simulink model "eovsa_corr_300mhz"  (R2012b)
settings: Solver=VariableStepDiscrete  SolverMode=SingleTasking  StartTime=0.0  StopTime=5000  RelTol=1e-3
undefined symbols (not defined in the file or in its folder): A, B, gcbh, PCIN, sfp, xlBlockLoadCallback, xlipgetpartsetting
libraries: xbsIndex_r4 x5996, casper_library_misc x52, simulink x33, dspsigops x24, xps_library x15, casper_library_delays x2
(part 7 of 65)

== system eovsa_corr_300mhz/pfb_fft ==
  note: If this register is not zero, the FFT
      | is overflowing, and you should change
      | the shift shedule to downshift more often.
  fft_shift : Inport
  acc_len : Inport  Port=2
  sync : Inport  Port=3
  adc0_pol0 : Inport  Port=4
  adc0_pol1 : Inport  Port=5
  adc1_pol0 : Inport  Port=6
  adc1_pol1 : Inport  Port=7
  acc_start_skip : Inport  Port=8
  clear_status : Inport  Port=9
  Constant : xbsIndex_r4/Constant  const=0  gui_display_data_type=Fixed-point  arith_type=Unsigned  n_bits=4  bin_pt=0  preci_type=Single  exp_width=8  frac_width=24  explicit_period=on  period=1  equ=P=C  opselect=C  inp2=PCIN>>17  opr=+  inp1=P  carry=CIN  dbl_ovrd=off  block_type=constant
  Convert : xbsIndex_r4/Convert  gui_display_data_type=Fixed-point  arith_type=Unsigned  n_bits=32  bin_pt=0  float_type=Single  exp_bits=8  fraction_bits=24  quantization=Truncate  overflow=Wrap  en=off  latency=0  dbl_ovrd=off  pipeline=off  block_type=convert
      settings: block_version=11.4
  Delay{6..7,12,19..20,24,34,42,47..48} (10 alike) : xbsIndex_r4/Delay  rst=off  infoeditControl=Selection of Reset will increase slice count due to use of real FFs and instead of SRLs  en=off  latency=2  dbl_ovrd=off  reg_retiming=on  block_type=delay
      settings: block_version=11.4
  Register : xbsIndex_r4/Register  init=0  rst=on  en=on  dbl_ovrd=off  block_type=register
  Relational : xbsIndex_r4/Relational  mode=a!=b  en=off  latency=0  dbl_ovrd=off  block_type=relational
  Terminator{10..16} (7 alike) : Terminator
  bus_expand : Subsystem  AncestorBlock=casper_library_flow_control/bus_expand  mask(bus_expand){mode=divisions of equal size, outputNum=4, outputWidth=12, outputBinaryPt=11, outputArithmeticType=1, show_format=off, outputToWorkspace=off, variablePrefix=out, outputToModelAsWell=on}
      mask prompts: outputNum "Number of outputs:"; outputWidth "Output width:"; outputBinaryPt "Output binary point position:"; outputArithmeticType "Output arithmetic type (ufix=0, fix=1, bool=2):"; show_format "Print format string?"; outputToWorkspace "Output to workspace?"; variablePrefix "Variable name prefix:"; outputToModelAsWell "Output to model as well?"
      mask help:
      | Expands a 'bus' made using a bus_create or Xilinx
      | concat block.
      | The input will be divided into the specified number
      | of outputs with the specified arithmetic types.
      | Divisions are made from most significant bit.
      mask init: same as eovsa_corr_300mhz/bus_expand7
      settings: AttributesFormatString=4 outputs
      mask TypeOptions mode: divisions of equal size | divisions of arbitrary size
      mask Callback mode: bus_expand_callback();
      mask Callback outputWidth: bus_expand_callback();
      mask Callback outputToWorkspace: bus_expand_callback();
  bus_expand1 : Subsystem  AncestorBlock=casper_library_flow_control/bus_expand  mask(bus_expand){mode=divisions of equal size, outputNum=4, outputWidth=12, outputBinaryPt=11, outputArithmeticType=1, show_format=off, outputToWorkspace=off, variablePrefix=out, outputToModelAsWell=on}
      mask prompts: outputNum "Number of outputs:"; outputWidth "Output width:"; outputBinaryPt "Output binary point position:"; outputArithmeticType "Output arithmetic type (ufix=0, fix=1, bool=2):"; show_format "Print format string?"; outputToWorkspace "Output to workspace?"; variablePrefix "Variable name prefix:"; outputToModelAsWell "Output to model as well?"
      mask help:
      | Expands a 'bus' made using a bus_create or Xilinx
      | concat block.
      | The input will be divided into the specified number
      | of outputs with the specified arithmetic types.
      | Divisions are made from most significant bit.
      mask init: same as eovsa_corr_300mhz/bus_expand7
      settings: AttributesFormatString=4 outputs
      mask TypeOptions mode: divisions of equal size | divisions of arbitrary size
      mask Callback mode: bus_expand_callback();
      mask Callback outputWidth: bus_expand_callback();
      mask Callback outputToWorkspace: bus_expand_callback();
  bus_expand2 : Subsystem  AncestorBlock=casper_library_flow_control/bus_expand  mask(bus_expand){mode=divisions of equal size, outputNum=4, outputWidth=12, outputBinaryPt=11, outputArithmeticType=1, show_format=off, outputToWorkspace=off, variablePrefix=out, outputToModelAsWell=on}
      mask prompts: outputNum "Number of outputs:"; outputWidth "Output width:"; outputBinaryPt "Output binary point position:"; outputArithmeticType "Output arithmetic type (ufix=0, fix=1, bool=2):"; show_format "Print format string?"; outputToWorkspace "Output to workspace?"; variablePrefix "Variable name prefix:"; outputToModelAsWell "Output to model as well?"
      mask help:
      | Expands a 'bus' made using a bus_create or Xilinx
      | concat block.
      | The input will be divided into the specified number
      | of outputs with the specified arithmetic types.
      | Divisions are made from most significant bit.
      mask init: same as eovsa_corr_300mhz/bus_expand7
      settings: AttributesFormatString=4 outputs
      mask TypeOptions mode: divisions of equal size | divisions of arbitrary size
      mask Callback mode: bus_expand_callback();
      mask Callback outputWidth: bus_expand_callback();
      mask Callback outputToWorkspace: bus_expand_callback();
  bus_expand3 : Subsystem  AncestorBlock=casper_library_flow_control/bus_expand  mask(bus_expand){mode=divisions of equal size, outputNum=4, outputWidth=12, outputBinaryPt=11, outputArithmeticType=1, show_format=off, outputToWorkspace=off, variablePrefix=out, outputToModelAsWell=on}
      mask prompts: outputNum "Number of outputs:"; outputWidth "Output width:"; outputBinaryPt "Output binary point position:"; outputArithmeticType "Output arithmetic type (ufix=0, fix=1, bool=2):"; show_format "Print format string?"; outputToWorkspace "Output to workspace?"; variablePrefix "Variable name prefix:"; outputToModelAsWell "Output to model as well?"
      mask help:
      | Expands a 'bus' made using a bus_create or Xilinx
      | concat block.
      | The input will be divided into the specified number
      | of outputs with the specified arithmetic types.
      | Divisions are made from most significant bit.
      mask init: same as eovsa_corr_300mhz/bus_expand7
      settings: AttributesFormatString=4 outputs
      mask TypeOptions mode: divisions of equal size | divisions of arbitrary size
      mask Callback mode: bus_expand_callback();
      mask Callback outputWidth: bus_expand_callback();
      mask Callback outputToWorkspace: bus_expand_callback();
  fft_wideband_real : xbsIndex_r4/Black Box  init_code=fft_wideband_real_core_config  sim_method=Inactive  verbose=off  block_type=blackbox2
      settings: block_version=11.4
  overflow : Subsystem  Tag=xps:sw_reg  AncestorBlock=xps_library/software_register  mask(swreg){mode=one value, io_dir=To Processor, io_delay=0, sample_period=1, names=reg, bitwidths=32, arith_types=0, bin_pts=0, sim_port=on, show_format=off}
      mask prompts: io_dir "I/O direction"; io_delay "I/O delay"; sample_period "Sample period"; names "Name:"; bitwidths "Bitwidth:"; arith_types "Type (ufix=0, fix=1, bool=2):"; bin_pts "Binary pt:"; sim_port "Provide sim input/output?"; show_format "Print format string?"
      mask init:
      | swreg_init(gcb)
      settings: AttributesFormatString=1output
      mask TypeOptions mode: one value | fields of equal size | fields of arbitrary size
      mask Callback mode: swreg_cb(gcb);
      mask TypeOptions io_dir: To Processor | From Processor
      mask Callback io_dir:
      | mask_enables = get_param(gcb, 'MaskEnables');
      | mask_names = get_param(gcb, 'MaskNames');
      | if strcmp(get_param(gcb, 'io_dir'), 'To Processor'),
      |     mask_enables{ismember(mask_names, 'sample_period')} = 'off';
      | else
      |     mask_enables{ismember(mask_names, 'sample_period')} = 'on';
      | end
      | set_param(gcb, 'MaskEnables', mask_enables);
      mask Callback bitwidths:
      | swreg_maskcheck(gcb);
      | % blk = gcb;
      | % mode = get_param(blk, 'mode');
      | % current_widths = eval(get_param(blk, 'bitwidths'));
      | % if (strcmp(mode, 'one value') || strcmp(mode, 'fields of equal size')) && (length(current_widths) > 1),
      | %     error('Only one width may be specified for this mode.');
      | % elseif strcmp(mode, 'fields of arbitrary size')
      | %     current_names = textscan(strtrim(strrep(strrep(get_param(blk, 'names'), ']', ''), '[', '')), '%s');
      | %     current_names = current_names{1};
      | %     numios = length(current_names);
      | %     if length(current_widths) ~= numios,
      | %         error('%d field names specified, but %d widths?', numios, length(current_widths));
      | %     end
      | % end
      | % total_width = 0;
      | % for ctr = 1 : length(current_widths),
      | %     total_width = total_width + current_widths(ctr);
      | % end
      | % if total_width > 32,
      | %     error('Total width must be 32 or less, set to %d.', total_width);
      | % end
      mask Callback arith_types:
      | [numios, ~, ~, ~, current_types] = swreg_maskcheck(gcb);
      | % blk = gcb;
      | % mode = get_param(blk, 'mode');
      | % current_types = eval(get_param(blk, 'arith_types'));
      | % numios = length(current_types);
      | % if (strcmp(mode, 'one value') || strcmp(mode, 'fields of equal size')) && (length(current_types) > 1),
      | %     error('Only one type may be specified for this mode.');
      | % elseif strcmp(mode, 'fields of arbitrary size')
      | %     current_names = textscan(strtrim(strrep(strrep(get_param(blk, 'names'), ']', ''), '[', '')), '%s');
      | %     current_names = current_names{1};
      | %     numios = length(current_names);
      | %     if length(current_types) ~= numios,
      | %         error('%d field names specified, but %d types?', numios, length(current_types));
      | %     end
      | % end
      | problem = 0;
      | for ctr = 1 : numios,
      |     t = current_types(ctr);
      |     if (t < 0) || (t > 2),
      |         problem = t;
      |         ctr = numios + 1;
      |     end
      | end
      | if problem ~= 0,
      |     error('Type cannot be %i, must be 0, 1 or 2.', problem);
      | end
      mask Callback bin_pts:
      | swreg_maskcheck(gcb);
      | % blk = gcb;
      | % mode = get_param(blk, 'mode');
      | % current_bins = eval(get_param(blk, 'bin_pts'));
      | % if (strcmp(mode, 'one value') || strcmp(mode, 'fields of equal size')) && (length(current_bins) > 1),
      | %     error('Only one binary pt may be specified for this mode.');
      | % elseif strcmp(mode, 'fields of arbitrary size')
      | %     current_names = textscan(strtrim(strrep(strrep(get_param(blk, 'names'), ']', ''), '[', '')), '%s');
      | %     current_names = current_names{1};
      | %     numios = length(current_names);
      | %     if length(current_bins) ~= numios,
      | %         error('%d field names specified, but %d binary pts?', numios, length(current_bins));
      | %     end
      | % end
  pfb_fir_real : xbsIndex_r4/Black Box  init_code=pfb_fir_4input_core_config  sim_method=Inactive  verbose=off  block_type=blackbox2
      settings: block_version=11.4
  power_td1 : Subsystem
  power_td2 : Subsystem
  power_td3 : Subsystem
  power_td4 : Subsystem
  sync_out0 : Outport
  x0_out0 : Outport  Port=2
  x0_out1 : Outport  Port=3
  y0_out0 : Outport  Port=4
  y0_out1 : Outport  Port=5
  x1_out0 : Outport  Port=6
  x1_out1 : Outport  Port=7
  y1_out0 : Outport  Port=8
  y1_out1 : Outport  Port=9
  adc0_pol0_P : Outport  Port=10
  adc0_pol0_P2 : Outport  Port=11
  adc0_pol1_P : Outport  Port=12
  adc0_pol1_P2 : Outport  Port=13
  adc1_pol0_P : Outport  Port=14
  adc1_pol0_P2 : Outport  Port=15
  adc1_pol1_P : Outport  Port=16
  adc1_pol1_P2 : Outport  Port=17
  acc_num : Outport  Port=18
  acc_valid : Outport  Port=19
  wires:
  power_td1/2(P) -> Delay47/1
  power_td1/3(P2) -> Delay48/1
  power_td1/4(acc_valid) -> Delay34/1
  [acc_start_skip] -> power_td1/4(acc_start_skip)
  acc_len/1 -> [acc_len]
  fft_wideband_real/10 -> Relational/1, Terminator13/1
  Relational/1 -> Register/3, Register/1
  Constant/1 -> Relational/2
  Register/1 -> Convert/1
  clear_status/1 -> Register/2
  Convert/1 -> overflow/1(out_reg)
  fft_shift/1 -> fft_wideband_real/2
  acc_start_skip/1 -> [acc_start_skip]
  sync/1 -> [sync], pfb_fir_real/1
  adc0_pol0/1 -> power_td1/2(din), pfb_fir_real/2
  adc0_pol1/1 -> power_td2/2(din), pfb_fir_real/3
  adc1_pol0/1 -> power_td3/2(din), pfb_fir_real/4
  adc1_pol1/1 -> power_td4/2(din), pfb_fir_real/5
  [acc_len] -> power_td1/3(acc_len)
  [sync] -> power_td1/1(sync)
  power_td2/2(P) -> Delay6/1
  power_td2/3(P2) -> Delay7/1
  power_td2/1(acc_num) -> Terminator10/1
  power_td2/4(acc_valid) -> Terminator11/1
  [acc_start_skip] -> power_td2/4(acc_start_skip)
  [acc_len] -> power_td2/3(acc_len)
  Delay6/1 -> adc0_pol1_P/1
  Delay7/1 -> adc0_pol1_P2/1
  [sync] -> power_td2/1(sync)
  power_td3/2(P) -> Delay12/1
  power_td3/3(P2) -> Delay19/1
  power_td3/1(acc_num) -> Terminator12/1
  power_td3/4(acc_valid) -> Terminator14/1
  [acc_start_skip] -> power_td3/4(acc_start_skip)
  [acc_len] -> power_td3/3(acc_len)
  [sync] -> power_td3/1(sync)
  power_td4/2(P) -> Delay20/1
  power_td4/3(P2) -> Delay24/1
  power_td4/1(acc_num) -> Terminator15/1
  power_td4/4(acc_valid) -> Terminator16/1
  [acc_start_skip] -> power_td4/4(acc_start_skip)
  [acc_len] -> power_td4/3(acc_len)
  Delay20/1 -> adc1_pol1_P/1
  Delay24/1 -> adc1_pol1_P2/1
  [sync] -> power_td4/1(sync)
  power_td1/1(acc_num) -> Delay42/1
  Delay12/1 -> adc1_pol0_P/1
  Delay19/1 -> adc1_pol0_P2/1
  Delay42/1 -> acc_num/1
  Delay47/1 -> adc0_pol0_P/1
  Delay48/1 -> adc0_pol0_P2/1
  Delay34/1 -> acc_valid/1
  pfb_fir_real/1 -> fft_wideband_real/1
  bus_expand/1(msb_out4) -> fft_wideband_real/3
  bus_expand/3(out2) -> fft_wideband_real/5
  bus_expand/2(out3) -> fft_wideband_real/4
  bus_expand/4(lsb_out1) -> fft_wideband_real/6
  bus_expand1/4(lsb_out1) -> fft_wideband_real/10
  bus_expand1/3(out2) -> fft_wideband_real/9
  bus_expand1/2(out3) -> fft_wideband_real/8
  bus_expand1/1(msb_out4) -> fft_wideband_real/7
  bus_expand2/2(out3) -> fft_wideband_real/12
  bus_expand2/1(msb_out4) -> fft_wideband_real/11
  bus_expand2/4(lsb_out1) -> fft_wideband_real/14
  bus_expand3/3(out2) -> fft_wideband_real/17
  bus_expand2/3(out2) -> fft_wideband_real/13
  bus_expand3/2(out3) -> fft_wideband_real/16
  bus_expand3/4(lsb_out1) -> fft_wideband_real/18
  bus_expand3/1(msb_out4) -> fft_wideband_real/15
  pfb_fir_real/2 -> bus_expand/1(bus_in)
  pfb_fir_real/3 -> bus_expand1/1(bus_in)
  pfb_fir_real/4 -> bus_expand2/1(bus_in)
  pfb_fir_real/5 -> bus_expand3/1(bus_in)
  fft_wideband_real/1 -> sync_out0/1
  fft_wideband_real/2 -> x0_out0/1
  fft_wideband_real/3 -> x0_out1/1
  fft_wideband_real/4 -> y0_out0/1
  fft_wideband_real/5 -> y0_out1/1
  fft_wideband_real/6 -> x1_out0/1
  fft_wideband_real/7 -> x1_out1/1
  fft_wideband_real/8 -> y1_out0/1
  fft_wideband_real/9 -> y1_out1/1

== system eovsa_corr_300mhz/phase_switching ==
  walsh_start : Inport
  phs_ant0 : Inport  Port=2
  phs_ant1 : Inport  Port=3
  adc0_0_0 : Inport  Port=4
  adc0_0_1 : Inport  Port=5
  adc0_0_2 : Inport  Port=6
  adc0_0_3 : Inport  Port=7
  adc0_1_0 : Inport  Port=8
  adc0_1_1 : Inport  Port=9
  adc0_1_2 : Inport  Port=10
  adc0_1_3 : Inport  Port=11
  adc0_sync : Inport  Port=12
  adc0_overflow : Inport  Port=13
  adc1_0_0 : Inport  Port=14
  adc1_0_1 : Inport  Port=15
  adc1_0_2 : Inport  Port=16
  adc1_0_3 : Inport  Port=17
  adc1_1_0 : Inport  Port=18
  adc1_1_1 : Inport  Port=19
  adc1_1_2 : Inport  Port=20
  adc1_1_3 : Inport  Port=21
  adc1_sync : Inport  Port=22
  adc1_overflow : Inport  Port=23
  pps_in : Inport  Port=24
  Delay{1,3..4,7,9,12,14..16,18} (10 alike) : xbsIndex_r4/Delay  rst=off  infoeditControl=Selection of Reset will increase slice count due to use of real FFs and instead of SRLs  en=off  latency=1  dbl_ovrd=off  reg_retiming=on  block_type=delay
  Delay{2,5,8,10..11,13,17} (7 alike) : xbsIndex_r4/Delay  rst=off  infoeditControl=Selection of Reset will increase slice count due to use of real FFs and instead of SRLs  en=off  latency=9  dbl_ovrd=off  reg_retiming=on  block_type=delay
  Delay6 : xbsIndex_r4/Delay  rst=off  infoeditControl=Selection of Reset will increase slice count due to use of real FFs and instead of SRLs  en=off  latency=10  dbl_ovrd=off  reg_retiming=on  block_type=delay
  Mux1 : xbsIndex_r4/Mux  inputs=2  en=off  latency=1  precision=Full  arith_type=Unsigned  n_bits=16  bin_pt=14  quantization=Truncate  overflow=Wrap  dbl_ovrd=off  block_type=mux
      settings: block_version=11.4
  phase_switching_select : Subsystem
  pol_pack0 : Subsystem
  pol_pack1 : Subsystem
  pol_pack2 : Subsystem
  pol_pack3 : Subsystem
  sync_out : Outport
  adc0_pol0 : Outport  Port=2
  adc0_pol1 : Outport  Port=3
  adc_sync : Outport  Port=4
  adc0_overflow_out : Outport  Port=5
  adc1_pol0 : Outport  Port=6
  adc1_pol1 : Outport  Port=7
  adc1_overflow_out : Outport  Port=8
  wires:
  pol_pack0/1(Out) -> Delay1/1
  pol_pack3/1(Out) -> Delay4/1
  phase_switching_select/2(phs_val_ant0) -> pol_pack0/1(phase), pol_pack3/1(phase)
  walsh_start/1 -> phase_switching_select/1(walsh_start)
  phase_switching_select/1(sync_out) -> Delay16/1
  Delay16/1 -> Delay15/1
  adc0_0_0/1 -> pol_pack0/2(In1)
  adc0_0_1/1 -> pol_pack0/3(In2)
  adc0_0_2/1 -> pol_pack0/4(In3)
  adc0_0_3/1 -> pol_pack0/5(In4)
  adc0_1_0/1 -> pol_pack3/2(In1)
  adc0_1_1/1 -> pol_pack3/3(In2)
  adc0_1_2/1 -> pol_pack3/4(In3)
  adc0_1_3/1 -> pol_pack3/5(In4)
  adc0_overflow/1 -> Delay3/1
  Delay3/1 -> Delay12/1
  pol_pack1/1(Out) -> Delay14/1
  pol_pack2/1(Out) -> Delay18/1
  phase_switching_select/3(phs_val_ant1) -> pol_pack2/1(phase), pol_pack1/1(phase)
  adc1_0_0/1 -> pol_pack1/2(In1)
  adc1_0_1/1 -> pol_pack1/3(In2)
  adc1_0_2/1 -> pol_pack1/4(In3)
  adc1_0_3/1 -> pol_pack1/5(In4)
  adc1_1_0/1 -> pol_pack2/2(In1)
  adc1_1_1/1 -> pol_pack2/3(In2)
  adc1_1_2/1 -> pol_pack2/4(In3)
  adc1_1_3/1 -> pol_pack2/5(In4)
  adc1_overflow/1 -> Delay7/1
  Delay7/1 -> Delay6/1
  Delay15/1 -> Delay8/1
  Delay6/1 -> adc1_overflow_out/1
  phs_ant0/1 -> phase_switching_select/2(ant_0_seq)
  phs_ant1/1 -> phase_switching_select/3(ant_1_seq)
  adc0_sync/1 -> Mux1/2
  adc1_sync/1 -> Mux1/3
  Mux1/1 -> Delay9/1
  Delay8/1 -> sync_out/1
  Delay1/1 -> Delay2/1
  Delay2/1 -> adc0_pol0/1
  Delay4/1 -> Delay5/1
  Delay5/1 -> adc0_pol1/1
  Delay9/1 -> Delay10/1
  Delay10/1 -> adc_sync/1
  Delay12/1 -> Delay11/1
  Delay11/1 -> adc0_overflow_out/1
  Delay14/1 -> Delay13/1
  Delay13/1 -> adc1_pol0/1
  Delay18/1 -> Delay17/1
  Delay17/1 -> adc1_pol1/1
  pps_in/1 -> Mux1/1

== system eovsa_corr_300mhz/pipeline21 ==
  d : Inport
  Register0 : xbsIndex_r4/Register  init=0  rst=off  en=off  dbl_ovrd=off  block_type=register
      settings: block_version=11.4
  q : Outport
  wires:
  d/1 -> Register0/1
  Register0/1 -> q/1

== system eovsa_corr_300mhz/pkt_gate ==
  rst_i : Inport
  data_i : Inport  Port=2
  dv_i : Inport  Port=3
  ip_i : Inport  Port=4
  port_i : Inport  Port=5
  eof_i : Inport  Port=6
  Delay25 : xbsIndex_r4/Delay  rst=off  infoeditControl=Selection of Reset will increase slice count due to use of real FFs and instead of SRLs  en=off  latency=1  dbl_ovrd=off  reg_retiming=off  block_type=delay
      settings: block_version=11.4
  Delay26 : xbsIndex_r4/Delay  rst=off  infoeditControl=Selection of Reset will increase slice count due to use of real FFs and instead of SRLs  en=off  latency=1  dbl_ovrd=off  reg_retiming=off  block_type=delay
      settings: block_version=11.4
  Delay27 : xbsIndex_r4/Delay  rst=off  infoeditControl=Selection of Reset will increase slice count due to use of real FFs and instead of SRLs  en=off  latency=1  dbl_ovrd=off  reg_retiming=on  block_type=delay
      settings: block_version=11.4
  Delay48 : xbsIndex_r4/Delay  rst=off  infoeditControl=Selection of Reset will increase slice count due to use of real FFs and instead of SRLs  en=off  latency=1  dbl_ovrd=off  reg_retiming=on  block_type=delay
      settings: block_version=11.4
  Delay49 : xbsIndex_r4/Delay  rst=off  infoeditControl=Selection of Reset will increase slice count due to use of real FFs and instead of SRLs  en=off  latency=1  dbl_ovrd=off  reg_retiming=on  block_type=delay
      settings: block_version=11.4
  Logical12 : xbsIndex_r4/Logical  logical_function=AND  inputs=2  en=off  latency=1  precision=Full  arith_type=Unsigned  n_bits=16  bin_pt=0  align_bp=on  dbl_ovrd=off  block_type=logical
  Register : xbsIndex_r4/Register  init=0  rst=off  en=on  dbl_ovrd=off  block_type=register
  rst_o : Outport
  data_o : Outport  Port=2
  dv_o : Outport  Port=3
  ip_o : Outport  Port=4
  port_o : Outport  Port=5
  eof_o : Outport  Port=6
  wires:
  rst_i/1 -> Delay26/1
  Delay26/1 -> rst_o/1
  Delay27/1 -> data_o/1
  data_i/1 -> Delay27/1
  port_i/1 -> Delay49/1
  eof_i/1 -> Register/2, Delay25/1
  dv_i/1 -> Logical12/2
  Delay49/1 -> port_o/1
  Delay25/1 -> eof_o/1
  ip_i/1 -> Delay48/1
  Logical12/1 -> dv_o/1
  Delay48/1 -> ip_o/1
  [ten_gbe_en] -> Register/1
  Register/1 -> Logical12/1

== system eovsa_corr_300mhz/pkt_gate1 ==
  rst_i : Inport
  data_i : Inport  Port=2
  dv_i : Inport  Port=3
  ip_i : Inport  Port=4
  port_i : Inport  Port=5
  eof_i : Inport  Port=6
  Delay{25..27,49} (4 alike) : xbsIndex_r4/Delay  rst=off  infoeditControl=Selection of Reset will increase slice count due to use of real FFs and instead of SRLs  en=off  latency=3  dbl_ovrd=off  reg_retiming=on  block_type=delay
      settings: block_version=11.4
  Delay48 : xbsIndex_r4/Delay  rst=off  infoeditControl=Selection of Reset will increase slice count due to use of real FFs and instead of SRLs  en=off  latency=0  dbl_ovrd=off  reg_retiming=on  block_type=delay
      settings: block_version=11.4
  Logical12 : xbsIndex_r4/Logical  logical_function=AND  inputs=2  en=off  latency=3  precision=Full  arith_type=Unsigned  n_bits=16  bin_pt=0  align_bp=on  dbl_ovrd=off  block_type=logical
  Register : xbsIndex_r4/Register  init=0  rst=off  en=on  dbl_ovrd=off  block_type=register
  rst_o : Outport
  data_o : Outport  Port=2
  dv_o : Outport  Port=3
  ip_o : Outport  Port=4
  port_o : Outport  Port=5
  eof_o : Outport  Port=6
  wires:
  rst_i/1 -> Delay26/1
  Delay26/1 -> rst_o/1
  Delay27/1 -> data_o/1
  data_i/1 -> Delay27/1
  port_i/1 -> Delay49/1
  eof_i/1 -> Register/2, Delay25/1
  dv_i/1 -> Logical12/2
  Delay49/1 -> port_o/1
  Delay25/1 -> eof_o/1
  ip_i/1 -> Delay48/1
  Logical12/1 -> dv_o/1
  Delay48/1 -> ip_o/1
  Register/1 -> Logical12/1
  [ten_gbe_en] -> Register/1

== system eovsa_corr_300mhz/pkt_gate2 ==
  rst_i : Inport
  data_i : Inport  Port=2
  dv_i : Inport  Port=3
  ip_i : Inport  Port=4
  port_i : Inport  Port=5
  eof_i : Inport  Port=6
  Delay{25..27,49} (4 alike) : xbsIndex_r4/Delay  rst=off  infoeditControl=Selection of Reset will increase slice count due to use of real FFs and instead of SRLs  en=off  latency=3  dbl_ovrd=off  reg_retiming=on  block_type=delay
      settings: block_version=11.4
  Delay48 : xbsIndex_r4/Delay  rst=off  infoeditControl=Selection of Reset will increase slice count due to use of real FFs and instead of SRLs  en=off  latency=0  dbl_ovrd=off  reg_retiming=on  block_type=delay
      settings: block_version=11.4
  Logical12 : xbsIndex_r4/Logical  logical_function=AND  inputs=2  en=off  latency=3  precision=Full  arith_type=Unsigned  n_bits=16  bin_pt=0  align_bp=on  dbl_ovrd=off  block_type=logical
  Register : xbsIndex_r4/Register  init=0  rst=off  en=on  dbl_ovrd=off  block_type=register
  rst_o : Outport
  data_o : Outport  Port=2
  dv_o : Outport  Port=3
  ip_o : Outport  Port=4
  port_o : Outport  Port=5
  eof_o : Outport  Port=6
  wires:
  [ten_gbe_en] -> Register/1
  Register/1 -> Logical12/1
  Delay48/1 -> ip_o/1
  Logical12/1 -> dv_o/1
  ip_i/1 -> Delay48/1
  Delay25/1 -> eof_o/1
  Delay49/1 -> port_o/1
  dv_i/1 -> Logical12/2
  eof_i/1 -> Delay25/1, Register/2
  port_i/1 -> Delay49/1
  data_i/1 -> Delay27/1
  Delay27/1 -> data_o/1
  Delay26/1 -> rst_o/1
  rst_i/1 -> Delay26/1

== system eovsa_corr_300mhz/pkt_gate3 ==
  rst_i : Inport
  data_i : Inport  Port=2
  dv_i : Inport  Port=3
  ip_i : Inport  Port=4
  port_i : Inport  Port=5
  eof_i : Inport  Port=6
  Delay{25..27,48..49} (5 alike) : xbsIndex_r4/Delay  rst=off  infoeditControl=Selection of Reset will increase slice count due to use of real FFs and instead of SRLs  en=off  latency=1  dbl_ovrd=off  reg_retiming=on  block_type=delay
      settings: block_version=11.4
  Logical12 : xbsIndex_r4/Logical  logical_function=AND  inputs=2  en=off  latency=1  precision=Full  arith_type=Unsigned  n_bits=16  bin_pt=0  align_bp=on  dbl_ovrd=off  block_type=logical
  Register : xbsIndex_r4/Register  init=0  rst=off  en=on  dbl_ovrd=off  block_type=register
  rst_o : Outport
  data_o : Outport  Port=2
  dv_o : Outport  Port=3
  ip_o : Outport  Port=4
  port_o : Outport  Port=5
  eof_o : Outport  Port=6
  wires:
  rst_i/1 -> Delay26/1
  Delay26/1 -> rst_o/1
  Delay27/1 -> data_o/1
  data_i/1 -> Delay27/1
  port_i/1 -> Delay49/1
  eof_i/1 -> Register/2, Delay25/1
  dv_i/1 -> Logical12/2
  Delay49/1 -> port_o/1
  Delay25/1 -> eof_o/1
  ip_i/1 -> Delay48/1
  Logical12/1 -> dv_o/1
  Delay48/1 -> ip_o/1
  Register/1 -> Logical12/1
  [ten_gbe_en] -> Register/1

== system eovsa_corr_300mhz/pol_snap ==
  note: Generate stop
      | when in circular
      | capture mode
  note: Delay start
      | of capture
  note: ctrl:
      | bit0: Put a posedge here
      |         to enable a new capture.
      | bit1: ignore external trigger
      |         and trigger immediately.
      | bit2: ignore external write
      |         enable and capture on
      |         every FPGA clock.
      | bit3: continuously capture
      |         data until we get an
      |         external stop command.
  note: Offset in vector
      | from first element
      | captured, used
      | during circular capture
  note: Number of
      | bytes in
      | buffer and
      | done bit
  note: Number of valid
      | data samples to
      | skip after trigger
      | before starting
      | capture
  note: Value on vin
      | aligned with
      | first sample on
      | din captured
  din : Inport
  we : Inport  Port=2
  trig : Inport  Port=3
  add_del : xbsIndex_r4/Delay  rst=off  infoeditControl=Selection of Reset will increase slice count due to use of real FFs and instead of SRLs  en=off  latency=1  dbl_ovrd=off  reg_retiming=on  block_type=delay
      settings: block_version=11.4
  add_gen : Subsystem  AncestorBlock=casper_library_scopes/snapshot/add_gen  mask{counter_size=11+3+1, increment=8, nsamples=11, burst_size=0, use_dsp48=on}
      mask prompts: counter_size "Address counter size (2^?)"; increment "Address counter increment"; nsamples "Number of samples (2^?)"; burst_size "Burst size (2^?)"; use_dsp48 "dsp48 counter/s"
      mask init:
      | set_param(gcb,'LinkStatus','inactive');
      | if strcmp(use_dsp48,'on'),
      |     set_param([gcb,'/add_gen'],'implementation','DSP48');
      | else
      |     set_param([gcb,'/add_gen'],'implementation','Fabric');
      | end
  basic_ctrl : Subsystem  AncestorBlock=casper_library_scopes/snapshot/basic_ctrl  mask{dram=off, data_width=64}
      mask prompts: data_width "data width"
  bram : Subsystem  Tag=xps:bram  AncestorBlock=xps_library/Shared BRAM  mask{arith_type=Unsigned, addr_width=11, data_width=64, reg_prim_output=on, reg_core_output=on, optimization=Minimum_Area, data_bin_pt=0, init_vals=[0:2^10-1], sample_rate=1}
      mask prompts: arith_type "Output Data Type"; addr_width "Address width"; data_width "Data Width"; reg_prim_output "Register Primitive Output"; reg_core_output "Register Core Output"; data_bin_pt "Data Binary Point"; init_vals "Initial values (simulation only)"; sample_rate "Sample rate"
      mask init:
      | shared_bram_mask;
      mask TypeOptions arith_type: Unsigned | Signed  (2's comp)
      mask TypeOptions data_width: 8 | 16 | 32 | 64 | 128
      mask TypeOptions optimization: Minimum_Area | Low_Power
  cast : xbsIndex_r4/Convert  gui_display_data_type=Fixed-point  arith_type=Unsigned  n_bits=64  bin_pt=0  float_type=Single  exp_bits=8  fraction_bits=24  quantization=Truncate  overflow=Wrap  en=off  latency=0  dbl_ovrd=off  pipeline=off  block_type=convert
      settings: block_version=11.4
  const0 : Constant  Value=0
  ctrl : Subsystem  Tag=xps:sw_reg  AncestorBlock=xps_library/software_register  mask(swreg){mode=one value, io_dir=From Processor, io_delay=0, sample_period=1, names=reg, bitwidths=32, arith_types=0, bin_pts=0, sim_port=on, show_format=off}
      mask prompts: io_dir "I/O direction"; io_delay "I/O delay"; sample_period "Sample period"; names "Name:"; bitwidths "Bitwidth:"; arith_types "Type (ufix=0, fix=1, bool=2):"; bin_pts "Binary pt:"; sim_port "Provide sim input/output?"; show_format "Print format string?"
      mask init:
      | swreg_init(gcb)
      settings: AttributesFormatString=1input
      mask TypeOptions mode: one value | fields of equal size | fields of arbitrary size
      mask Callback mode: swreg_cb(gcb);
      mask TypeOptions io_dir: To Processor | From Processor
      mask Callback io_dir:
      | mask_enables = get_param(gcb, 'MaskEnables');
      | mask_names = get_param(gcb, 'MaskNames');
      | if strcmp(get_param(gcb, 'io_dir'), 'To Processor'),
      |     mask_enables{ismember(mask_names, 'sample_period')} = 'off';
      | else
      |     mask_enables{ismember(mask_names, 'sample_period')} = 'on';
      | end
      | set_param(gcb, 'MaskEnables', mask_enables);
      mask Callback bitwidths:
      | swreg_maskcheck(gcb);
      | % blk = gcb;
      | % mode = get_param(blk, 'mode');
      | % current_widths = eval(get_param(blk, 'bitwidths'));
      | % if (strcmp(mode, 'one value') || strcmp(mode, 'fields of equal size')) && (length(current_widths) > 1),
      | %     error('Only one width may be specified for this mode.');
      | % elseif strcmp(mode, 'fields of arbitrary size')
      | %     current_names = textscan(strtrim(strrep(strrep(get_param(blk, 'names'), ']', ''), '[', '')), '%s');
      | %     current_names = current_names{1};
      | %     numios = length(current_names);
      | %     if length(current_widths) ~= numios,
      | %         error('%d field names specified, but %d widths?', numios, length(current_widths));
      | %     end
      | % end
      | % total_width = 0;
      | % for ctr = 1 : length(current_widths),
      | %     total_width = total_width + current_widths(ctr);
      | % end
      | % if total_width > 32,
      | %     error('Total width must be 32 or less, set to %d.', total_width);
      | % end
      mask Callback arith_types:
      | [numios, ~, ~, ~, current_types] = swreg_maskcheck(gcb);
      | % blk = gcb;
      | % mode = get_param(blk, 'mode');
      | % current_types = eval(get_param(blk, 'arith_types'));
      | % numios = length(current_types);
      | % if (strcmp(mode, 'one value') || strcmp(mode, 'fields of equal size')) && (length(current_types) > 1),
      | %     error('Only one type may be specified for this mode.');
      | % elseif strcmp(mode, 'fields of arbitrary size')
      | %     current_names = textscan(strtrim(strrep(strrep(get_param(blk, 'names'), ']', ''), '[', '')), '%s');
      | %     current_names = current_names{1};
      | %     numios = length(current_names);
      | %     if length(current_types) ~= numios,
      | %         error('%d field names specified, but %d types?', numios, length(current_types));
      | %     end
      | % end
      | problem = 0;
      | for ctr = 1 : numios,
      |     t = current_types(ctr);
      |     if (t < 0) || (t > 2),
      |         problem = t;
      |         ctr = numios + 1;
      |     end
      | end
      | if problem ~= 0,
      |     error('Type cannot be %i, must be 0, 1 or 2.', problem);
      | end
      mask Callback bin_pts:
      | swreg_maskcheck(gcb);
      | % blk = gcb;
      | % mode = get_param(blk, 'mode');
      | % current_bins = eval(get_param(blk, 'bin_pts'));
      | % if (strcmp(mode, 'one value') || strcmp(mode, 'fields of equal size')) && (length(current_bins) > 1),
      | %     error('Only one binary pt may be specified for this mode.');
      | % elseif strcmp(mode, 'fields of arbitrary size')
      | %     current_names = textscan(strtrim(strrep(strrep(get_param(blk, 'names'), ']', ''), '[', '')), '%s');
      | %     current_names = current_names{1};
      | %     numios = length(current_names);
      | %     if length(current_bins) ~= numios,
      | %         error('%d field names specified, but %d binary pts?', numios, length(current_bins));
      | %     end
      | % end
  dat_del : xbsIndex_r4/Delay  rst=off  infoeditControl=Selection of Reset will increase slice count due to use of real FFs and instead of SRLs  en=off  latency=1  dbl_ovrd=off  reg_retiming=off  block_type=delay
      settings: block_version=11.4
  g_tr_en_cnt : Terminator
  gbram : Terminator
  gstatus : Terminator
  gval : Terminator
  never : xbsIndex_r4/Constant  const=0  gui_display_data_type=Fixed-point  arith_type=Boolean  n_bits=16  bin_pt=14  preci_type=Single  exp_width=8  frac_width=24  explicit_period=on  period=1  equ=P=C  opselect=C  inp2=PCIN>>17  opr=+  inp1=P  carry=CIN  dbl_ovrd=off  block_type=constant
  ri : xbsIndex_r4/Reinterpret  force_arith_type=on  arith_type=Unsigned  force_bin_pt=on  bin_pt=0  block_type=reinterpret
      settings: infoedit="Changes signal type without altering the binary representation.   You can changed the signal between signed and unsigned, and relocate the binary point.<br><br>Hardware notes: In hardware this block costs nothing.<br><br>Example:  Suppose the input is 6 bits wide, signed, with 2 fractional bits, and the output is forced to unsigned with 0 fractional bits.  Then an input of -2.0 (1110.00 in binary 2's complement) becomes an output of 56 (111000 in binary)."
  status : Subsystem  Tag=xps:sw_reg  AncestorBlock=xps_library/software_register  mask(swreg){mode=one value, io_dir=To Processor, io_delay=0, sample_period=1, names=reg, bitwidths=32, arith_types=0, bin_pts=0, sim_port=on, show_format=off}
      mask prompts: io_dir "I/O direction"; io_delay "I/O delay"; sample_period "Sample period"; names "Name:"; bitwidths "Bitwidth:"; arith_types "Type (ufix=0, fix=1, bool=2):"; bin_pts "Binary pt:"; sim_port "Provide sim input/output?"; show_format "Print format string?"
      mask init:
      | swreg_init(gcb)
      settings: AttributesFormatString=1output
      mask TypeOptions mode: one value | fields of equal size | fields of arbitrary size
      mask Callback mode: swreg_cb(gcb);
      mask TypeOptions io_dir: To Processor | From Processor
      mask Callback io_dir:
      | mask_enables = get_param(gcb, 'MaskEnables');
      | mask_names = get_param(gcb, 'MaskNames');
      | if strcmp(get_param(gcb, 'io_dir'), 'To Processor'),
      |     mask_enables{ismember(mask_names, 'sample_period')} = 'off';
      | else
      |     mask_enables{ismember(mask_names, 'sample_period')} = 'on';
      | end
      | set_param(gcb, 'MaskEnables', mask_enables);
      mask Callback bitwidths:
      | swreg_maskcheck(gcb);
      | % blk = gcb;
      | % mode = get_param(blk, 'mode');
      | % current_widths = eval(get_param(blk, 'bitwidths'));
      | % if (strcmp(mode, 'one value') || strcmp(mode, 'fields of equal size')) && (length(current_widths) > 1),
      | %     error('Only one width may be specified for this mode.');
      | % elseif strcmp(mode, 'fields of arbitrary size')
      | %     current_names = textscan(strtrim(strrep(strrep(get_param(blk, 'names'), ']', ''), '[', '')), '%s');
      | %     current_names = current_names{1};
      | %     numios = length(current_names);
      | %     if length(current_widths) ~= numios,
      | %         error('%d field names specified, but %d widths?', numios, length(current_widths));
      | %     end
      | % end
      | % total_width = 0;
      | % for ctr = 1 : length(current_widths),
      | %     total_width = total_width + current_widths(ctr);
      | % end
      | % if total_width > 32,
      | %     error('Total width must be 32 or less, set to %d.', total_width);
      | % end
      mask Callback arith_types:
      | [numios, ~, ~, ~, current_types] = swreg_maskcheck(gcb);
      | % blk = gcb;
      | % mode = get_param(blk, 'mode');
      | % current_types = eval(get_param(blk, 'arith_types'));
      | % numios = length(current_types);
      | % if (strcmp(mode, 'one value') || strcmp(mode, 'fields of equal size')) && (length(current_types) > 1),
      | %     error('Only one type may be specified for this mode.');
      | % elseif strcmp(mode, 'fields of arbitrary size')
      | %     current_names = textscan(strtrim(strrep(strrep(get_param(blk, 'names'), ']', ''), '[', '')), '%s');
      | %     current_names = current_names{1};
      | %     numios = length(current_names);
      | %     if length(current_types) ~= numios,
      | %         error('%d field names specified, but %d types?', numios, length(current_types));
      | %     end
      | % end
      | problem = 0;
      | for ctr = 1 : numios,
      |     t = current_types(ctr);
      |     if (t < 0) || (t > 2),
      |         problem = t;
      |         ctr = numios + 1;
      |     end
      | end
      | if problem ~= 0,
      |     error('Type cannot be %i, must be 0, 1 or 2.', problem);
      | end
      mask Callback bin_pts:
      | swreg_maskcheck(gcb);
      | % blk = gcb;
      | % mode = get_param(blk, 'mode');
      | % current_bins = eval(get_param(blk, 'bin_pts'));
      | % if (strcmp(mode, 'one value') || strcmp(mode, 'fields of equal size')) && (length(current_bins) > 1),
      | %     error('Only one binary pt may be specified for this mode.');
      | % elseif strcmp(mode, 'fields of arbitrary size')
      | %     current_names = textscan(strtrim(strrep(strrep(get_param(blk, 'names'), ']', ''), '[', '')), '%s');
      | %     current_names = current_names{1};
      | %     numios = length(current_names);
      | %     if length(current_bins) ~= numios,
      | %         error('%d field names specified, but %d binary pts?', numios, length(current_bins));
      | %     end
      | % end
  vin_const : xbsIndex_r4/Constant  const=0  gui_display_data_type=Fixed-point  arith_type=Boolean  n_bits=16  bin_pt=14  preci_type=Single  exp_width=8  frac_width=24  explicit_period=on  period=1  equ=P=C  opselect=C  inp2=PCIN>>17  opr=+  inp1=P  carry=CIN  dbl_ovrd=off  block_type=constant
  we_del : xbsIndex_r4/Delay  rst=off  infoeditControl=Selection of Reset will increase slice count due to use of real FFs and instead of SRLs  en=off  latency=1  dbl_ovrd=off  reg_retiming=on  block_type=delay
      settings: block_version=11.4
  wires:
  din/1 -> ri/1
  ri/1 -> cast/1
  cast/1 -> basic_ctrl/2(din)
  we/1 -> basic_ctrl/3(we)
  trig/1 -> basic_ctrl/4(trig)
  never/1 -> basic_ctrl/6(stopi)
  const0/1 -> ctrl/1(sim_1)
  ctrl/1(in_reg) -> basic_ctrl/5(ctrl)
  basic_ctrl/1(vout) -> add_gen/1(vin)
  basic_ctrl/2(dout) -> add_gen/2(din)
  basic_ctrl/3(we_o) -> add_gen/3(we)
  basic_ctrl/4(go) -> add_gen/4(go)
  basic_ctrl/5(stop) -> add_gen/5(cont)
  basic_ctrl/6(init) -> add_gen/6(init)
  add_gen/5(status) -> status/1(out_reg)
  status/1(sim_out) -> gstatus/1
  vin_const/1 -> basic_ctrl/1(vin)
  add_gen/1(vout) -> gval/1
  add_gen/6(en_cnt) -> g_tr_en_cnt/1
  add_gen/2(add) -> add_del/1
  add_gen/3(dout) -> dat_del/1
  add_gen/4(we_o) -> we_del/1
  add_del/1 -> bram/1(addr)
  dat_del/1 -> bram/2(data_in)
  we_del/1 -> bram/3(we)
  bram/1(data_out) -> gbram/1

== system eovsa_corr_300mhz/power_cal ==
  sync_in : Inport
  pol1_f0 : Inport  Port=2
  pol1_f1 : Inport  Port=3
  pol2_f0 : Inport  Port=4
  pol2_f1 : Inport  Port=5
  pol3_f0 : Inport  Port=6
  pol3_f1 : Inport  Port=7
  pol4_f0 : Inport  Port=8
  pol4_f1 : Inport  Port=9
  Delay4 : xbsIndex_r4/Delay  rst=off  infoeditControl=Selection of Reset will increase slice count due to use of real FFs and instead of SRLs  en=off  latency=13  dbl_ovrd=off  reg_retiming=on  block_type=delay
      settings: xl_area=[0, 0, 0, 0, 0, 0, 0]  block_version=10.1.2
  power_full1 : Subsystem
  power_full2 : Subsystem
  power_full3 : Subsystem
  power_full4 : Subsystem
  power_full5 : Subsystem
  power_full6 : Subsystem
  power_full7 : Subsystem
  power_full8 : Subsystem
  sync_out : Outport
  pol1_f0_pow : Outport  Port=2
  pol1_f1_pow : Outport  Port=3
  pol2_f0_pow : Outport  Port=4
  pol2_f1_pow : Outport  Port=5
  pol3_f0_pow : Outport  Port=6
  pol3_f1_pow : Outport  Port=7
  pol4_f0_pow : Outport  Port=8
  pol4_f1_pow : Outport  Port=9
  pol1_f0_pow_sq : Outport  Port=10
  pol1_f1_pow_sq : Outport  Port=11
  pol2_f0_pow_sq : Outport  Port=12
  pol2_f1_pow_sq : Outport  Port=13
  pol3_f0_pow_sq : Outport  Port=14
  pol3_f1_pow_sq : Outport  Port=15
  pol4_f0_pow_sq : Outport  Port=16
  pol4_f1_pow_sq : Outport  Port=17
  wires:
  sync_in/1 -> Delay4/1
  pol1_f0/1 -> power_full6/1(c)
  pol1_f1/1 -> power_full1/1(c)
  pol2_f0/1 -> power_full3/1(c)
  pol2_f1/1 -> power_full2/1(c)
  pol3_f0/1 -> power_full4/1(c)
  pol3_f1/1 -> power_full7/1(c)
  pol4_f0/1 -> power_full5/1(c)
  pol4_f1/1 -> power_full8/1(c)
  power_full6/1(power) -> pol1_f0_pow/1
  power_full6/2(power_sq) -> pol1_f0_pow_sq/1
  power_full1/1(power) -> pol1_f1_pow/1
  power_full1/2(power_sq) -> pol1_f1_pow_sq/1
  power_full3/1(power) -> pol2_f0_pow/1
  power_full3/2(power_sq) -> pol2_f0_pow_sq/1
  power_full2/1(power) -> pol2_f1_pow/1
  power_full2/2(power_sq) -> pol2_f1_pow_sq/1
  power_full4/1(power) -> pol3_f0_pow/1
  power_full4/2(power_sq) -> pol3_f0_pow_sq/1
  power_full7/1(power) -> pol3_f1_pow/1
  power_full7/2(power_sq) -> pol3_f1_pow_sq/1
  power_full5/1(power) -> pol4_f0_pow/1
  power_full5/2(power_sq) -> pol4_f0_pow_sq/1
  power_full8/1(power) -> pol4_f1_pow/1
  power_full8/2(power_sq) -> pol4_f1_pow_sq/1
  Delay4/1 -> sync_out/1

== system eovsa_corr_300mhz/pulse generator1 ==
  note: pulse goes high 3 clocks after sync
  sync : Inport
  Constant : xbsIndex_r4/Constant  const=0  gui_display_data_type=Fixed-point  arith_type=Unsigned  n_bits=ceil( log2( period - 1 ) )  bin_pt=0  preci_type=Single  exp_width=8  frac_width=24  explicit_period=on  period=1  equ=P=C  opselect=C  inp2=PCIN>>17  opr=+  inp1=P  carry=CIN  dbl_ovrd=off  block_type=constant
      settings: block_version=11.4
  Counter : xbsIndex_r4/Counter  cnt_type=Free Running  cnt_to=period - 1  operation=Up  start_count=0  cnt_by_val=1  arith_type=Unsigned  n_bits=ceil( log2 (period - 1))  bin_pt=0  load_pin=off  rst=on  en=off  explicit_period=on  period=1  dbl_ovrd=off  use_behavioral_HDL=on  implementation=DSP48  block_type=counter
      settings: block_version=11.4
  Logical : xbsIndex_r4/Logical  logical_function=AND  inputs=2  en=off  latency=1  precision=Full  arith_type=Unsigned  n_bits=16  bin_pt=0  align_bp=on  dbl_ovrd=off  block_type=logical
      settings: block_version=11.4
  Register : xbsIndex_r4/Register  init=0  rst=off  en=on  dbl_ovrd=off  block_type=register
      settings: block_version=11.4
  Register1 : xbsIndex_r4/Register  init=0  rst=off  en=off  dbl_ovrd=off  block_type=register
      settings: block_version=11.4
  Relational : xbsIndex_r4/Relational  mode=a=b  en=off  latency=1  dbl_ovrd=off  block_type=relational
  pulse : Outport
  wires:
  Register1/1 -> Logical/1
  Register/1 -> Register1/1
  Relational/1 -> Logical/2
  Constant/1 -> Relational/2
  Counter/1 -> Relational/1
  Logical/1 -> pulse/1
  sync/1 -> Register/2, Register/1, Counter/1

== system eovsa_corr_300mhz/pulse generator2 ==
  sync : Inport
  Constant : xbsIndex_r4/Constant  const=period - 3  gui_display_data_type=Fixed-point  arith_type=Unsigned  n_bits=ceil( log2( period - 1 ) )  bin_pt=0  preci_type=Single  exp_width=8  frac_width=24  explicit_period=on  period=1  equ=P=C  opselect=C  inp2=PCIN>>17  opr=+  inp1=P  carry=CIN  dbl_ovrd=off  block_type=constant
      settings: block_version=11.4
  Counter : xbsIndex_r4/Counter  cnt_type=Count Limited  cnt_to=period - 1  operation=Up  start_count=0  cnt_by_val=1  arith_type=Unsigned  n_bits=ceil( log2 (period - 1))  bin_pt=0  load_pin=off  rst=on  en=off  explicit_period=on  period=1  dbl_ovrd=off  use_behavioral_HDL=off  implementation=Fabric  block_type=counter
      settings: block_version=11.4
  Logical : xbsIndex_r4/Logical  logical_function=AND  inputs=2  en=off  latency=1  precision=Full  arith_type=Unsigned  n_bits=16  bin_pt=0  align_bp=on  dbl_ovrd=off  block_type=logical
      settings: block_version=11.4
  Logical1 : xbsIndex_r4/Logical  logical_function=OR  inputs=2  en=off  latency=0  precision=Full  arith_type=Unsigned  n_bits=16  bin_pt=0  align_bp=on  dbl_ovrd=off  block_type=logical
      settings: block_version=11.4
  Register : xbsIndex_r4/Register  init=0  rst=off  en=on  dbl_ovrd=off  block_type=register
      settings: block_version=11.4
  Register1 : xbsIndex_r4/Register  init=0  rst=off  en=off  dbl_ovrd=off  block_type=register
      settings: block_version=11.4
  Relational : xbsIndex_r4/Relational  mode=a=b  en=off  latency=1  dbl_ovrd=off  block_type=relational
  pulse : Outport
  wires:
  sync/1 -> Counter/1, Register/1, Register/2, Logical1/2
  Logical1/1 -> pulse/1
  Counter/1 -> Relational/1
  Constant/1 -> Relational/2
  Relational/1 -> Logical/2
  Logical/1 -> Logical1/1
  Register/1 -> Register1/1
  Register1/1 -> Logical/1

== system eovsa_corr_300mhz/pulse generator3 ==
  sync : Inport
  Constant : xbsIndex_r4/Constant  const=period - 3  gui_display_data_type=Fixed-point  arith_type=Unsigned  n_bits=ceil( log2( period - 1 ) )  bin_pt=0  preci_type=Single  exp_width=8  frac_width=24  explicit_period=on  period=1  equ=P=C  opselect=C  inp2=PCIN>>17  opr=+  inp1=P  carry=CIN  dbl_ovrd=off  block_type=constant
      settings: block_version=11.4
  Counter : xbsIndex_r4/Counter  cnt_type=Count Limited  cnt_to=period - 1  operation=Up  start_count=0  cnt_by_val=1  arith_type=Unsigned  n_bits=ceil( log2 (period - 1))  bin_pt=0  load_pin=off  rst=on  en=off  explicit_period=on  period=1  dbl_ovrd=off  use_behavioral_HDL=off  implementation=Fabric  block_type=counter
      settings: block_version=11.4
  Logical : xbsIndex_r4/Logical  logical_function=AND  inputs=2  en=off  latency=1  precision=Full  arith_type=Unsigned  n_bits=16  bin_pt=0  align_bp=on  dbl_ovrd=off  block_type=logical
      settings: block_version=11.4
  Logical1 : xbsIndex_r4/Logical  logical_function=OR  inputs=2  en=off  latency=0  precision=Full  arith_type=Unsigned  n_bits=16  bin_pt=0  align_bp=on  dbl_ovrd=off  block_type=logical
      settings: block_version=11.4
  Register : xbsIndex_r4/Register  init=0  rst=off  en=on  dbl_ovrd=off  block_type=register
      settings: block_version=11.4
  Register1 : xbsIndex_r4/Register  init=0  rst=off  en=off  dbl_ovrd=off  block_type=register
      settings: block_version=11.4
  Relational : xbsIndex_r4/Relational  mode=a=b  en=off  latency=1  dbl_ovrd=off  block_type=relational
  pulse : Outport
  wires:
  sync/1 -> Counter/1, Register/1, Register/2, Logical1/2
  Logical1/1 -> pulse/1
  Counter/1 -> Relational/1
  Constant/1 -> Relational/2
  Relational/1 -> Logical/2
  Logical/1 -> Logical1/1
  Register/1 -> Register1/1
  Register1/1 -> Logical/1
